simulink model "separetly_excited_DC_motor"  (R2021a)
settings: Solver=VariableStepAuto  StartTime=0.0  StopTime=100  RelTol=1e-3
values from neighbouring files (symbols this model uses):
  B = 0.01    [model_for_SEDC.m]
  J = 5    [model_for_SEDC.m]
  kphi = 1.6    [model_for_SEDC.m]
  La = 0.1    [model_for_SEDC.m]
  Ra = 0.5    [model_for_SEDC.m]
libraries: spsThyristorLib x4, spsVoltageMeasurementLib x3, spsACVoltageSourceLib x1, spspowerguiLib x1, spsSeriesRLCBranchLib x1, dspswit3 x1, spsUniversalBridgeLib x1
settings Model: Creator=YasserNet  LastModifiedBy=YasserNet

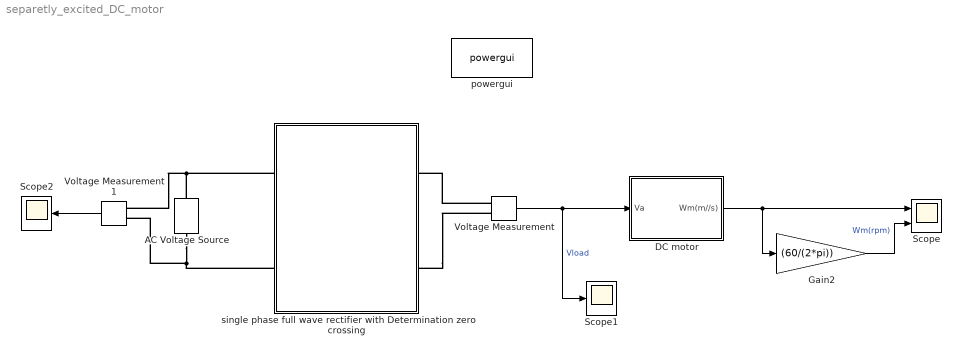
== system separetly_excited_DC_motor ==
  AC Voltage Source : spsACVoltageSourceLib/AC Voltage Source  Amplitude=220*sqrt(2)  Phase=0  Frequency=50  SampleTime=0  Measurements=None  BusType=swing  Pref=10e3  Qref=0  Qmin=-inf  Qmax=+inf
  DC motor : Subsystem
  Gain2 : Gain  Gain=(60/(2*pi))
  Scope : Scope  NumInputPorts=2
  Scope1 : Scope
  Scope2 : Scope
  Voltage Measurement : spsVoltageMeasurementLib/Voltage Measurement  PhasorSimulation=off  OutputType=Complex  PSBequivalent=0
  Voltage Measurement1 : spsVoltageMeasurementLib/Voltage Measurement  PhasorSimulation=off  OutputType=Complex  PSBequivalent=0
  powergui : spspowerguiLib/powergui  Priority=1  SimulationMode=Continuous  SampleTime=50e-6  frequency=60  Iterations=50  frequencyindice=50  Pbase=100e6  ErrMax=1e-4  UnitsV=kV  UnitsW=MW  buscounter=0  FunctionMessages=off  echomessages=off  EnableUseOfTLC=off  CurrentSourceSwitches=off  DisableSnubberDevices=off  DisableRonSwitches=off  DisableVfSwitches=off  DisplayEquations=off  AutomaticDiscreteSolvers=off  SolverType=Tustin/Backward Euler (TBE)  Interpol=off  ExternalGateDelay=off  methode=off  Ts=100  x0status=blocks  SPID=on  SwTol=0  HookPort=off  NonlinearTolerance=1e-4  nMaxIteration=100  ContinueOnMaxIteration=off  RestoreLinks=warning  ResistiveCurrentMeasurement=off  Frange=[0:2:500]  Ylog=off  Xlog=on  ShowGrid=off  save=off  variable=ZData  structure=0  ZoomFFT=off  StartTime=0.0  cycles=1  DisplayStyle=1  fundamental=60  FreqAxis=off  MaxFrequency=1000  frequencyindicesteady=1  RmsSteady=1  display=off
  "single phase full wave rectifier with Determination zero crossing " : Subsystem
  wires:
  Gain2/1 -> Scope/2  "Wm(rpm)"
  DC motor/1(Wm(m//s)) -> Scope/1, Gain2/1
  Voltage Measurement/1 -> DC motor/1(Va), Scope1/1  "Vload"
  Voltage Measurement1/1 -> Scope2/1
  connections:
  AC Voltage Source/RConn1 -- Voltage Measurement1/LConn2 -- "single phase full wave rectifier with Determination zero crossing "/LConn1
  AC Voltage Source/LConn1 -- Voltage Measurement1/LConn1 -- "single phase full wave rectifier with Determination zero crossing "/LConn2
  Voltage Measurement/LConn1 -- "single phase full wave rectifier with Determination zero crossing "/RConn1
  Voltage Measurement/LConn2 -- "single phase full wave rectifier with Determination zero crossing "/RConn2

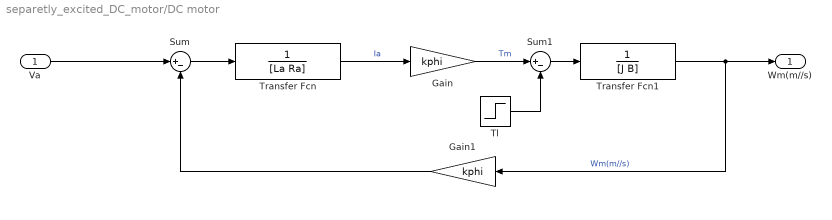
== system separetly_excited_DC_motor/DC motor ==
  Va : Inport
  Gain : Gain  Gain=kphi
  Gain1 : Gain  Gain=kphi
  Sum : Sum  Inputs=|+-
  Sum1 : Sum  Inputs=|+-
  Tl : Step  Time=6  Before=25  After=75  SampleTime=0
  Transfer Fcn : TransferFcn  Denominator=[La Ra]
  Transfer Fcn1 : TransferFcn  Denominator=[J B]
  Wm(m//s) : Outport
  wires:
  Transfer Fcn/1 -> Gain/1  "Ia"
  Tl/1 -> Sum1/2
  Gain/1 -> Sum1/1  "Tm"
  Sum1/1 -> Transfer Fcn1/1
  Transfer Fcn1/1 -> Wm(m//s)/1, Gain1/1  "Wm(m//s)"
  Sum/1 -> Transfer Fcn/1
  Gain1/1 -> Sum/2
  Va/1 -> Sum/1

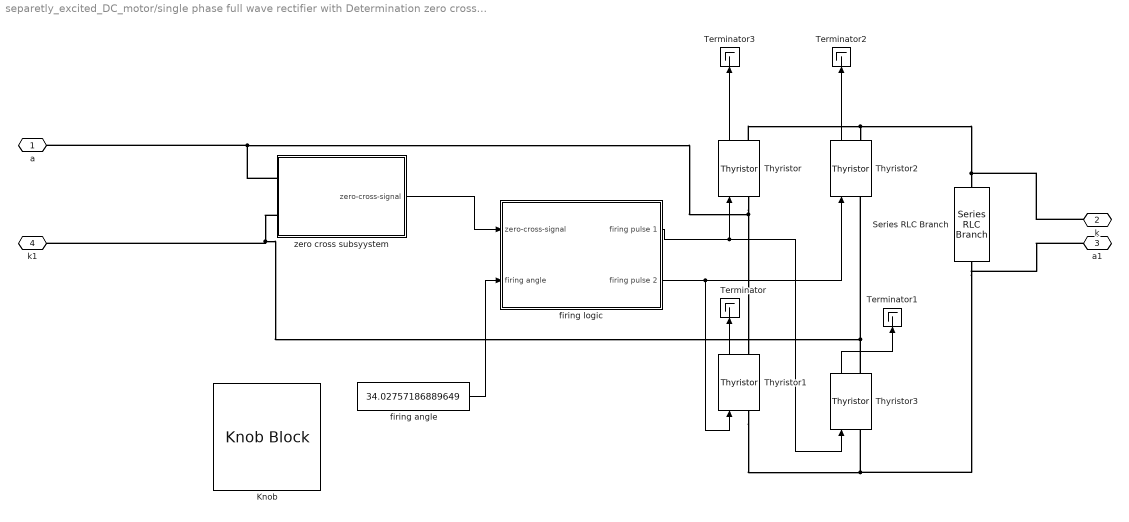
== system separetly_excited_DC_motor/single phase full wave rectifier with Determination zero crossing  ==
  Knob : KnobBlock  ScaleMax=180
  Series RLC Branch : spsSeriesRLCBranchLib/Series RLC Branch  LConnTagsString=__new0  RConnTagsString=__new0  BranchType=C  Resistance=1  Inductance=1e-3  SetiL0=off  InitialCurrent=0  Capacitance=1e-6  Setx0=off  InitialVoltage=0  Measurements=None
  Terminator{,1..3} (4 alike) : Terminator
  Thyristor{,1..3} (4 alike) : spsThyristorLib/Thyristor  Ron=0.001  Lon=0  Vf=0.8  IC=0  Rs=500  Cs=250e-9  Measurements=on
  firing angle : Constant  Value=34.02757186889649
  firing logic : Subsystem
  zero cross subsyystem : Subsystem
  a : PMIOPort  Side=Left
  k : PMIOPort  Port=2  Side=Right
  a1 : PMIOPort  Port=3  Side=Right
  k1 : PMIOPort  Port=4  Side=Left
  wires:
  zero cross subsyystem/1(zero-cross-signal) -> firing logic/1(zero-cross-signal)
  Thyristor1/1 -> Terminator/1
  Thyristor/1 -> Terminator3/1
  Thyristor3/1 -> Terminator1/1
  firing logic/2(firing pulse 2) -> Thyristor1/1, Thyristor2/1
  firing angle/1 -> firing logic/2(firing angle)
  firing logic/1(firing pulse 1) -> Thyristor/1, Thyristor3/1
  Thyristor2/1 -> Terminator2/1
  connections:
  Thyristor/RConn1 -- k/RConn1 -- Series RLC Branch/LConn1 -- Thyristor2/RConn1
  Thyristor1/LConn1 -- a1/RConn1 -- Series RLC Branch/RConn1 -- Thyristor3/LConn1
  zero cross subsyystem/LConn2 -- k1/RConn1 -- Thyristor2/LConn1 -- Thyristor3/RConn1
  zero cross subsyystem/LConn1 -- a/RConn1 -- Thyristor1/RConn1 -- Thyristor/LConn1

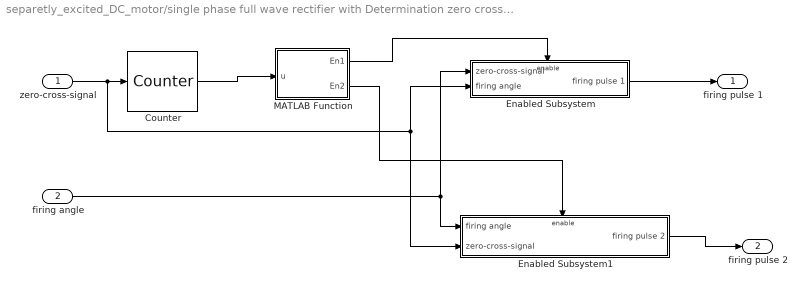
== system separetly_excited_DC_motor/single phase full wave rectifier with Determination zero crossing /firing logic ==
  zero-cross-signal : Inport
  firing angle : Inport  Port=2
  Counter : dspswit3/Counter  Direction=Up  CountEvent=Rising edge  CounterSize=User defined  MaxCount=255  InitialCount=0  Output=Count  HitValue=32  ResetInput=off  SamplesPerFrame=1  Ts=1  CntDtype=double  HitDtype=Logical
  Enabled Subsystem : Subsystem  TreatAsAtomicUnit=on
  Enabled Subsystem1 : Subsystem  TreatAsAtomicUnit=on
  MATLAB Function : MATLAB Function  TreatAsAtomicUnit=on
  firing pulse 1 : Outport
  firing pulse 2 : Outport  Port=2
  wires:
  zero-cross-signal/1 -> Enabled Subsystem/2(firing angle), Enabled Subsystem1/2(zero-cross-signal), Counter/1
  Counter/1 -> MATLAB Function/1(u)
  MATLAB Function/1(En1) -> Enabled Subsystem/Enable
  firing angle/1 -> Enabled Subsystem/1(zero-cross-signal), Enabled Subsystem1/1(firing angle)
  Enabled Subsystem/1(firing pulse 1) -> firing pulse 1/1
  Enabled Subsystem1/1(firing pulse 2) -> firing pulse 2/1
  MATLAB Function/2(En2) -> Enabled Subsystem1/Enable

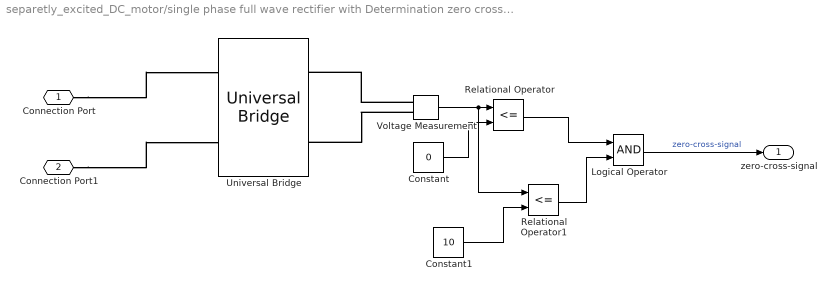
== system separetly_excited_DC_motor/single phase full wave rectifier with Determination zero crossing /zero cross subsyystem ==
  Constant : Constant  Value=0
  Constant1 : Constant  Value=10
  Logical Operator : Logic  AllPortsSameDT=off  OutDataTypeStr=boolean
  Relational Operator : RelationalOperator  Operator=<=  OutDataTypeStr=boolean  RndMeth=Simplest
  Relational Operator1 : RelationalOperator  Operator=<=  OutDataTypeStr=boolean  RndMeth=Simplest
  Universal Bridge : spsUniversalBridgeLib/Universal Bridge  Arms=2  SnubberResistance=1e5  SnubberCapacitance=inf  Device=Diodes  Ron=1e-3  Lon=0  ForwardVoltages="[  0  0  ]"  ForwardVoltage=0  GTOparameters=[ 10e-6 , 20e-6 ]  IGBTparameters=[ 1e-6 , 2e-6 ]  Measurements=None  Measurements_2=None  converterType=Rectifier
  Voltage Measurement : spsVoltageMeasurementLib/Voltage Measurement  PhasorSimulation=off  OutputType=Complex  PSBequivalent=0
  Connection Port : PMIOPort  Side=Left
  Connection Port1 : PMIOPort  Port=2  Side=Left
  zero-cross-signal : Outport
  wires:
  Voltage Measurement/1 -> Relational Operator1/1, Relational Operator/1
  Constant/1 -> Relational Operator/2
  Constant1/1 -> Relational Operator1/2
  Relational Operator/1 -> Logical Operator/1
  Relational Operator1/1 -> Logical Operator/2
  Logical Operator/1 -> zero-cross-signal/1  "zero-cross-signal"
  connections:
  Connection Port/RConn1 -- Universal Bridge/LConn1
  Connection Port1/RConn1 -- Universal Bridge/LConn2
  Voltage Measurement/LConn1 -- Universal Bridge/RConn1
  Voltage Measurement/LConn2 -- Universal Bridge/RConn2

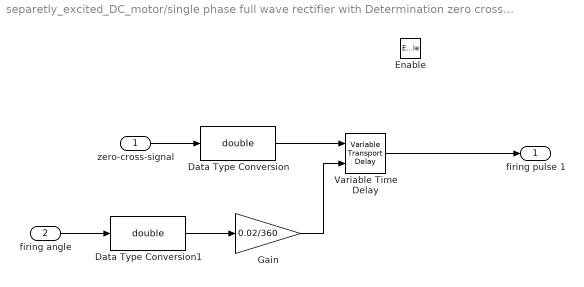
== system separetly_excited_DC_motor/single phase full wave rectifier with Determination zero crossing /firing logic/Enabled Subsystem ==
  zero-cross-signal : Inport
  firing angle : Inport  Port=2
  Enable : EnablePort
  Data Type Conversion : DataTypeConversion  OutDataTypeStr=double
  Data Type Conversion1 : DataTypeConversion  OutDataTypeStr=double
  Gain : Gain  Gain=0.02/360  OutDataTypeStr=double
  Variable Time Delay : VariableTransportDelay  MaximumDelay=10  MaximumPoints=13312  ZeroDelay=on
  firing pulse 1 : Outport
  wires:
  zero-cross-signal/1 -> Data Type Conversion/1
  Data Type Conversion/1 -> Variable Time Delay/1
  firing angle/1 -> Data Type Conversion1/1
  Gain/1 -> Variable Time Delay/2
  Variable Time Delay/1 -> firing pulse 1/1
  Data Type Conversion1/1 -> Gain/1

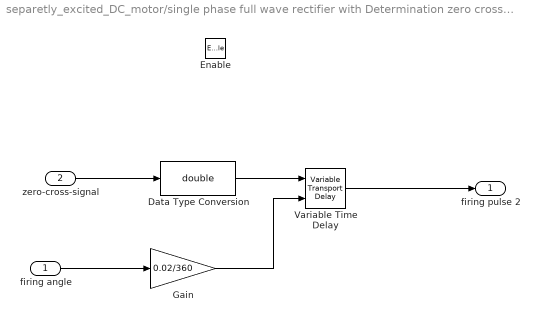
== system separetly_excited_DC_motor/single phase full wave rectifier with Determination zero crossing /firing logic/Enabled Subsystem1 ==
  firing angle : Inport
  zero-cross-signal : Inport  Port=2
  Enable : EnablePort
  Data Type Conversion : DataTypeConversion  OutDataTypeStr=double
  Gain : Gain  Gain=0.02/360
  Variable Time Delay : VariableTransportDelay  MaximumDelay=10
  firing pulse 2 : Outport
  wires:
  Data Type Conversion/1 -> Variable Time Delay/1
  Gain/1 -> Variable Time Delay/2
  Variable Time Delay/1 -> firing pulse 2/1
  zero-cross-signal/1 -> Data Type Conversion/1
  firing angle/1 -> Gain/1

== matlab function separetly_excited_DC_motor/single phase full wave rectifier with Determination zero crossing /firing logic/MATLAB Function ==
  data: u input; En1 output; En2 output
function [En1,En2] = fcn(u)
En1=0;
En2=0;
if mod(u,2)==0
En1=1;
En2=0;
end
if mod(u,2)==1
En1=0;
En2=1;
end
y = u;
